simulink model "Dynamic_articulation_FSFI"  (R2018b)
settings: Solver=VariableStepAuto  StartTime=0.0  StopTime=500  RelTol=1e-9
values from neighbouring files (symbols this model uses):
  A = [0 -1 0 0 0 0 0 0 ... (first row only)    [Dynamic_model_articulation.m]    (also in articulation1.m = E_matrix)
  a2 = input(12)    [Nonlinear_model.m]    (also in linear_model.m; linear_model_error.m; trailer_constants.m = 4.98)
  B1 = [0,B1(1),0,B1(2),0,B1(3),0,B1(4)]'    [articulation1.m]
  B2 = [0,B2(1),0,B2(2),0,B2(3),0,B2(4)]'    [articulation1.m]
  h1 = input(10)    [Nonlinear_model.m]    (also in linear_model.m; linear_model_error.m; truck_constants.m = 1.1)
  K = place(A,B1,Poles)    [FullStateFeedback.m]    (also in articulation.m = [(C+C3),     (Cs1-C3*(h1+l2)+(m1+m2)*u^2),    (-C3*l2),    (; articulation1.m = [(C+C3),     (Cs1-C3*(h1+l2)+(m1+m2)*u^2),    (-C3*l2),    (; linear_model.m = -1/u*K*x_bar; linear_model_error.m = -1/u*K*x_bar)
  Vx = 20    [Dynamic_model_articulation.m]
settings Model: Creator=kevingasik  LastModifiedBy=kevingasik
settings SolverCC: ConsecutiveZCsStepRelTol=100*128*eps  MaxConsecutiveMinStep=10

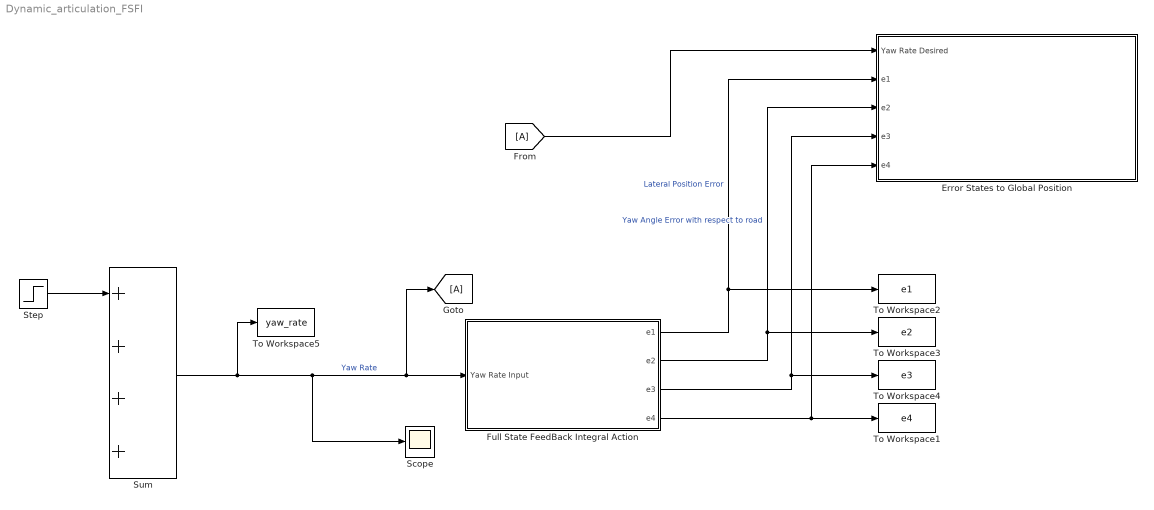
== system Dynamic_articulation_FSFI ==
  Error States to Global Position : Subsystem
  Full State FeedBack Integral Action : Subsystem
  Scope : Scope
  Step : Step  SampleTime=0
  Sum : Sum  Inputs=++++
  To Workspace1 : ToWorkspace  VariableName=e4  SampleTime=-1
      settings: Save2DSignal=2-D array (concatenate along first dimension)
  To Workspace2 : ToWorkspace  VariableName=e1  SampleTime=-1
      settings: Save2DSignal=2-D array (concatenate along first dimension)
  To Workspace3 : ToWorkspace  VariableName=e2  SampleTime=-1
      settings: Save2DSignal=2-D array (concatenate along first dimension)
  To Workspace4 : ToWorkspace  VariableName=e3  SampleTime=-1
      settings: Save2DSignal=2-D array (concatenate along first dimension)
  To Workspace5 : ToWorkspace  VariableName=yaw_rate  SampleTime=-1
      settings: Save2DSignal=2-D array (concatenate along first dimension)
  wires:
  Sum/1 -> To Workspace5/1, Full State FeedBack Integral Action/1(Yaw Rate Input), [A], Scope/1  "Yaw Rate"
  Full State FeedBack Integral Action/2(e2) -> Error States to Global Position/3(" e2"), To Workspace3/1  "Yaw Angle Error with respect to road"
  Full State FeedBack Integral Action/1(e1) -> Error States to Global Position/2(e1), To Workspace2/1  "Lateral Position Error"
  Full State FeedBack Integral Action/3(e3) -> Error States to Global Position/4(e3), To Workspace4/1
  Full State FeedBack Integral Action/4(e4) -> To Workspace1/1, Error States to Global Position/5(e4)
  Step/1 -> Sum/1
  [A] -> Error States to Global Position/1(Yaw Rate Desired)

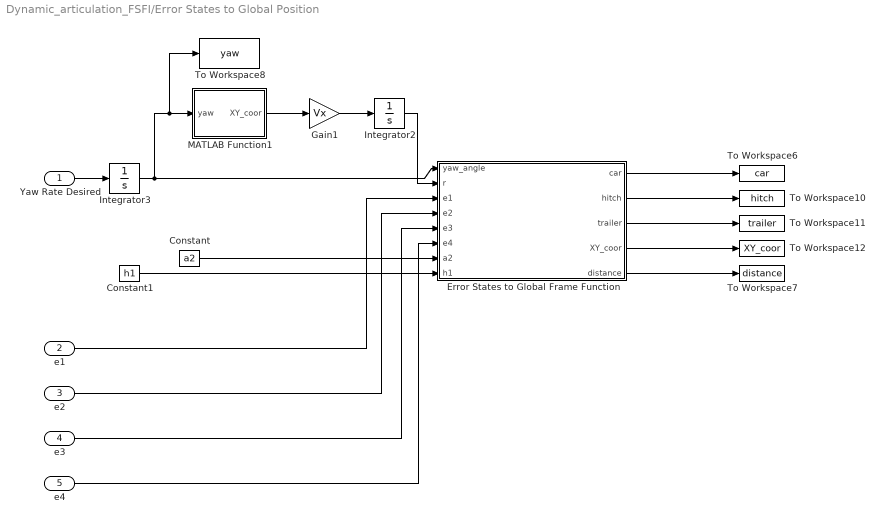
== system Dynamic_articulation_FSFI/Error States to Global Position ==
  Yaw Rate Desired : Inport
  e1 : Inport  Port=2
  " e2" : Inport  Port=3
  e3 : Inport  Port=4
  e4 : Inport  Port=5
  Constant : Constant  Value=a2
  Constant1 : Constant  Value=h1
  Error States to Global Frame Function : MATLAB Function  TreatAsAtomicUnit=on
  Gain1 : Gain  Gain=Vx
  Integrator2 : Integrator
  Integrator3 : Integrator
  MATLAB Function1 : MATLAB Function  TreatAsAtomicUnit=on
  To Workspace10 : ToWorkspace  VariableName=hitch  SampleTime=-1
      settings: Save2DSignal=2-D array (concatenate along first dimension)
  To Workspace11 : ToWorkspace  VariableName=trailer  SampleTime=-1
      settings: Save2DSignal=2-D array (concatenate along first dimension)
  To Workspace12 : ToWorkspace  VariableName=XY_coor  SampleTime=-1
      settings: Save2DSignal=2-D array (concatenate along first dimension)
  To Workspace6 : ToWorkspace  VariableName=car  SampleTime=-1
      settings: Save2DSignal=2-D array (concatenate along first dimension)
  To Workspace7 : ToWorkspace  VariableName=distance  SampleTime=-1
      settings: Save2DSignal=2-D array (concatenate along first dimension)
  To Workspace8 : ToWorkspace  VariableName=yaw  SampleTime=-1
      settings: Save2DSignal=2-D array (concatenate along first dimension)
  wires:
  e4/1 -> Error States to Global Frame Function/6(e4)
  " e2"/1 -> Error States to Global Frame Function/4(e2)
  e3/1 -> Error States to Global Frame Function/5(e3)
  Error States to Global Frame Function/2(hitch) -> To Workspace10/1
  Error States to Global Frame Function/4(XY_coor) -> To Workspace12/1
  Yaw Rate Desired/1 -> Integrator3/1
  Integrator3/1 -> To Workspace8/1, MATLAB Function1/1(yaw), Error States to Global Frame Function/1(yaw_angle)
  e1/1 -> Error States to Global Frame Function/3(e1)
  Integrator2/1 -> Error States to Global Frame Function/2(r)
  Error States to Global Frame Function/5(distance) -> To Workspace7/1
  Error States to Global Frame Function/3(trailer) -> To Workspace11/1
  Constant1/1 -> Error States to Global Frame Function/8(h1)
  Error States to Global Frame Function/1(car) -> To Workspace6/1
  Gain1/1 -> Integrator2/1
  Constant/1 -> Error States to Global Frame Function/7(a2)
  MATLAB Function1/1(XY_coor) -> Gain1/1

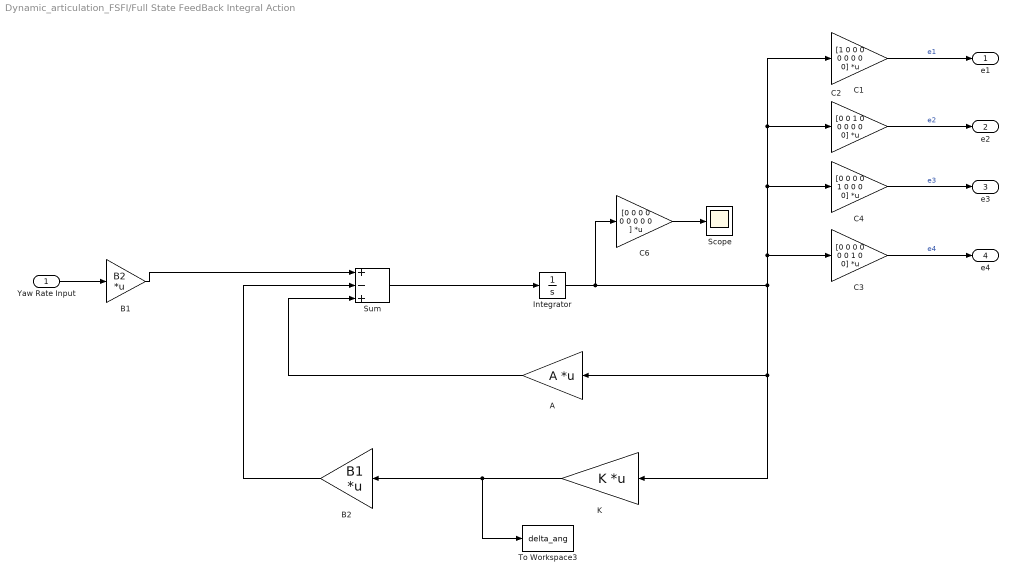
== system Dynamic_articulation_FSFI/Full State FeedBack Integral Action ==
  Yaw Rate Input : Inport
  A : Gain  Gain=A  Multiplication=Matrix(K*u)
  B1 : Gain  Gain=B2  Multiplication=Matrix(K*u)
  B2 : Gain  Gain=B1  Multiplication=Matrix(K*u)
  C1 : Gain  Gain=[1 0 0 0 0 0 0 0 0]  Multiplication=Matrix(K*u)
  C2 : Gain  Gain=[0 0 1 0 0 0 0 0 0]  Multiplication=Matrix(K*u)
  C3 : Gain  Gain=[0 0 0 0 0 0 1 0 0]  Multiplication=Matrix(K*u)
  C4 : Gain  Gain=[0 0 0 0 1 0 0 0 0]  Multiplication=Matrix(K*u)
  C6 : Gain  Gain=[0 0 0 0 0 0 0 0 0 ]  Multiplication=Matrix(K*u)
  Integrator : Integrator  InitialCondition=0.0001
  K : Gain  Gain=K  Multiplication=Matrix(K*u)
  Scope : Scope
  Sum : Sum  Inputs=|+-+
  To Workspace3 : ToWorkspace  VariableName=delta_ang  SampleTime=-1
      settings: Save2DSignal=2-D array (concatenate along first dimension)
  e1 : Outport
  e2 : Outport  Port=2
  e3 : Outport  Port=3
  e4 : Outport  Port=4
  wires:
  K/1 -> To Workspace3/1, B2/1
  Sum/1 -> Integrator/1
  C2/1 -> e2/1  "e2"
  Integrator/1 -> K/1, A/1, C4/1, C2/1, C1/1, C3/1, C6/1
  A/1 -> Sum/3
  B2/1 -> Sum/2
  B1/1 -> Sum/1
  C1/1 -> e1/1  "e1"
  C4/1 -> e3/1  "e3"
  C3/1 -> e4/1  "e4"
  Yaw Rate Input/1 -> B1/1
  C6/1 -> Scope/1

== matlab function Dynamic_articulation_FSFI/Error States to Global Position/Error States to Global Frame Function ==
  data: yaw_angle input; r input; e1 input; car output; hitch output; trailer output; XY_coor output; e2 input; e3 input; e4 input; a2 input; h1 input; distance output
function [car,hitch,trailer,XY_coor,distance] = fcn(yaw_angle,r,e1,e2,e3, e4, a2,h1)
XY_coor = [0 0];
trailer = [0 0];
hitch = [0 0];
car = [0 0];


%%Transformation matrices from local to global coordinates
Q = [-sind(yaw_angle+e2),cosd(yaw_angle+e2)];
R = [-cosd(yaw_angle+e2),-sind(yaw_angle+e2)];
T = [-cosd(yaw_angle+e4),-sind(yaw_angle+e4)];

%% desired trajectory
X_des = r(1,1);
Y_des = r(1,2);
%X_des2 = r(1,1) - (a2+h1)*cosd(yaw_angle+e2);
%Y_des2 = r(1,2) - (a2+h1)*sind(yaw_angle+e2);
XY_coor = [X_des,Y_des];

%outputting the correct output.
car_x = r(1,1)+ e1*Q(1,1);
car_y = r(1,2)+ e1*Q(1,2);
car = [car_x,car_y];

hitch_x = r(1,1) + e1*Q(1,1) + h1*R(1,1);
hitch_y = r(1,2) + e1*Q(1,2) + h1*R(1,2);
%hitch_a = X_des2 + e3*Q(1,1) - a2*T(1,1);
%hitch_b = Y_des2 + e3*Q(1,2) - a2*T(1,2);
hitch = [hitch_x,hitch_y];


trailer_x = r(1,1)+ (e1)*Q(1,1) + h1*R(1,1) + a2*T(1,1);
trailer_y = r(1,2)+ (e1)*Q(1,2) + h1*R(1,2) + a2*T(1,2);
%trailer_x = X_des2 + e3*Q(1,1);
%trailer_y = Y_des2 + e3*Q(1,2);
distance = sqrt((abs(hitch_x-trailer_x))^2 + abs(hitch_y-trailer_y)^2);
trailer = [trailer_x,trailer_y];

== matlab function Dynamic_articulation_FSFI/Error States to Global Position/MATLAB Function1 ==
  data: yaw input; XY_coor output
function XY_coor  = fcn(yaw)

XY_coor = [cosd(yaw),sind(yaw)];
